simulink subsystem "Data_Analysis"  (R2021b)
settings: Solver=VariableStepAuto  StartTime=0.0  StopTime=10.0  RelTol=1e-3
undefined symbols (not defined in the file or in its folder): Setpoint
settings Model: Creator=jsagardu  LastModifiedBy=jsagardu

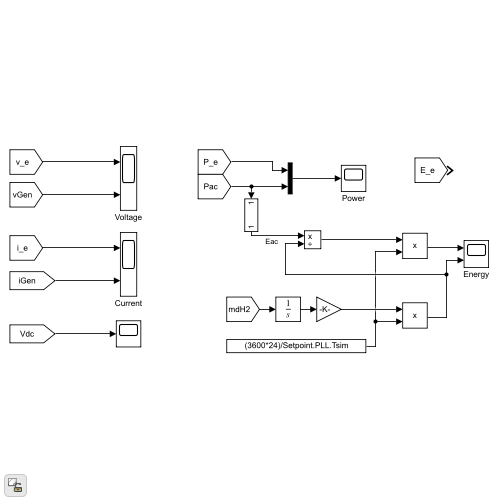
[thumbnail: Simulink's stored preview of the top-level diagram]
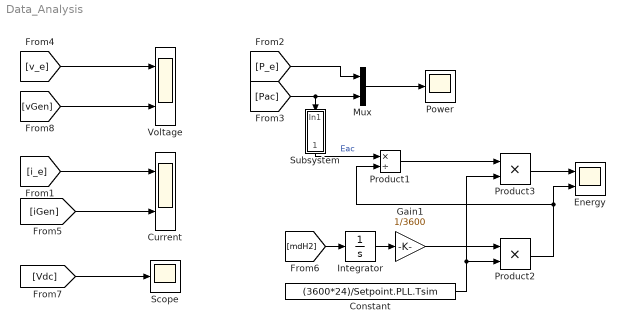
== system Data_Analysis ==
  Constant : Constant  Value=(3600*24)/Setpoint.PLL.Tsim
  Current : Scope  NumInputPorts=2
  Energy : Scope  NumInputPorts=2
  Gain1 : Gain  Gain=1/3600
  Integrator : Integrator
  Mux : Mux  Inputs=2
  Power : Scope
  Product1 : Product  Inputs=*/
  Product2 : Product  Inputs=**
  Product3 : Product  Inputs=**
  Scope : Scope
  Subsystem : Subsystem
  Voltage : Scope  NumInputPorts=2
  wires:
  [i_e] -> Current/1
  [iGen] -> Current/2
  [vGen] -> Voltage/2
  [P_e] -> Mux/1
  Mux/1 -> Power/1
  [v_e] -> Voltage/1
  [mdH2] -> Integrator/1
  Integrator/1 -> Gain1/1
  Product1/1 -> Product3/1
  Gain1/1 -> Product2/1
  Constant/1 -> Product3/2, Product2/2
  Product3/1 -> Energy/1
  Product2/1 -> Energy/2, Product1/2
  [Vdc] -> Scope/1
  Subsystem/1(Out1) -> Product1/1  "Eac"
  [Pac] -> Mux/2, Subsystem/1(In1)

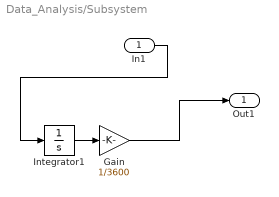
== system Data_Analysis/Subsystem ==
  In1 : Inport
  Gain : Gain  Gain=1/3600
  Integrator1 : Integrator
  Out1 : Outport
  wires:
  Gain/1 -> Out1/1
  In1/1 -> Integrator1/1
  Integrator1/1 -> Gain/1
